simulink model "sprawko3"  (R2019b)
settings: Solver=VariableStepAuto  StartTime=0.0  StopTime=10.0  RelTol=1e-3
values from neighbouring files (symbols this model uses):
  b = 2    [anal_c_d.m]    (also in symulacyjne3B.m)
undefined symbols (not defined in the file or in its folder): a, c, k
settings Model: Creator=margr  LastModifiedBy=margr

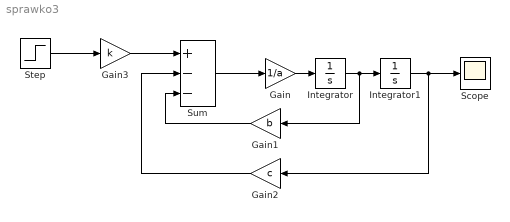
== system sprawko3 ==
  Gain : Gain  Gain=1/a
  Gain1 : Gain  Gain=b
  Gain2 : Gain  Gain=c
  Gain3 : Gain  Gain=k
  Integrator : Integrator
  Integrator1 : Integrator  InitialCondition=2
  Scope : Scope
  Step : Step  SampleTime=0
  Sum : Sum  Inputs=+--
  wires:
  Sum/1 -> Gain/1
  Gain/1 -> Integrator/1
  Integrator/1 -> Gain1/1, Integrator1/1
  Integrator1/1 -> Gain2/1, Scope/1
  Gain1/1 -> Sum/3
  Gain2/1 -> Sum/2
  Gain3/1 -> Sum/1
  Step/1 -> Gain3/1
